simulink model "dc_motor_5hp_model2"  (R2022a)
settings: Solver=ode45  StartTime=0.0  StopTime=6  RelTol=1e-3  EnableMultiTasking=on
values from neighbouring files (symbols this model uses):
  Dm = 1e-4    (= 0.0001)    [dc_par.m]    (also in dcm_par.m = 6.04e-06)
  J = 1    [dc_par.m]    (also in dcm_par.m = 2.12e-06)
  La = 0.012    [dc_par.m]    (also in dcm_par.m = 0.12)
  Laf = 1.8    [dc_par.m]    (also in dcm_par.m = 0.0395)
  Lf = 120    [dc_par.m]
  Ra = 0.6    [dc_par.m]    (also in dcm_par.m = 7)
  Rf = 240    [dc_par.m]
  Tm = 29    [dc_par.m]    (also in dcm_par.m = 0.00353)
  Va = 240    [dc_par.m]    (also in dcm_par.m = 6)
settings Model: Creator=Jurij  LastModifiedBy=Juri
settings SolverCC: AlgebraicLoopSolver=TrustRegion
settings DataIOCC: LimitDataPoints=on  MaxDataPoints=10000  SaveFormat=Array  SignalLoggingSaveFormat=ModelDataLogs  SaveOutput=off  SaveState=on  ReturnWorkspaceOutputs=off  StateSaveName=x  TimeSaveName=t  SignalLoggingName=sigsOut
settings OptimizationCC: LifeSpan=inf
settings DebuggingCC: SaveWithParameterizedLinksMsg=none  UnderspecifiedInitializationDetection=Classic  MergeDetectMultiDrivingBlocksExec=none  SignalResolutionControl=TryResolveAllWithWarning  MultiTaskDSMMsg=warning  MultiTaskCondExecSysMsg=none  UnconnectedInputMsg=warning  UnconnectedOutputMsg=warning  UnconnectedLineMsg=warning  SFUnexpectedBacktrackingDiag=warning  SFNoUnconditionalDefaultTransitionDiag=warning  SFExecutionAtInitializationDiag=none  SFMachineParentedDataDiag=warning  ArithmeticOperatorsInVariantConditions=warning
settings HardwareCC: ProdBitPerPointer=32  ProdBitPerSizeT=32  ProdBitPerPtrDiffT=32  ProdLargestAtomicFloat=None  ProdIntDivRoundTo=Undefined  ProdEndianess=Unspecified  ProdWordSize=32  ProdHWDeviceType=32-bit Generic  TargetUnknown=on
settings ModelReferenceCC: PropagateSignalLabelsOutOfModel=off
settings SFSimCC: SimUseLocalCustomCode=off  CustomCodeUndefinedFunction=UseInterfaceOnly
settings RTWCC: RTWUseLocalCustomCode=off
settings CodeAppCC: StateflowObjectComments=on
settings GRTTargetCC: TargetLangStandard=C89/C90 (ANSI)  CombineOutputUpdateFcns=off  GRTInterface=on
settings ConfigComp: CovMetricSettings=dw  CovSaveCumulativeToWorkspaceVar=on  CovSaveSingleToWorkspaceVar=on  CovExternalEMLEnable=off

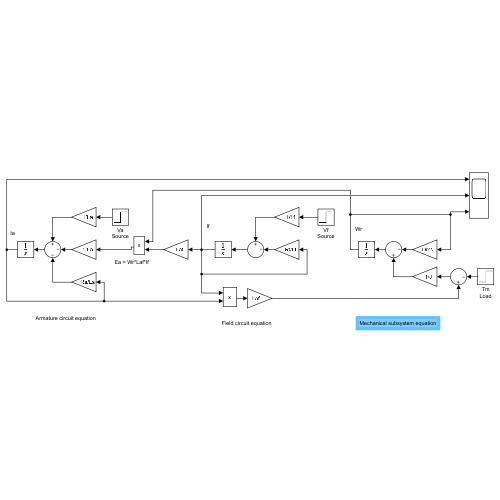
[thumbnail: Simulink's stored preview of the top-level diagram]
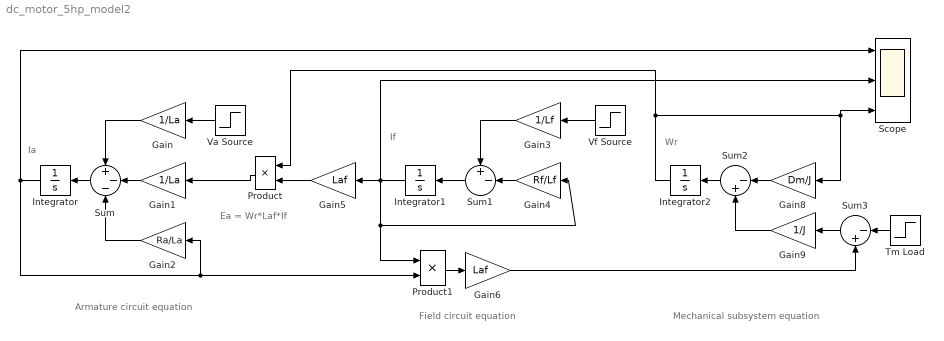
== system dc_motor_5hp_model2 ==
  note: Ia
  note: If
  note: Ea = Wr*Laf*If
  note: Wr
  note: Armature circuit equation
  note: Field circuit equation
  note: Mechanical subsystem equation
  Gain : Gain  Gain=1/La  SaturateOnIntegerOverflow=on  OutDataTypeStr=Inherit: Same as input  ParamDataTypeStr=Inherit: Same as input
  Gain1 : Gain  Gain=1/La  SaturateOnIntegerOverflow=on  OutDataTypeStr=Inherit: Same as input  ParamDataTypeStr=Inherit: Same as input
  Gain2 : Gain  Gain=Ra/La  SaturateOnIntegerOverflow=on  OutDataTypeStr=Inherit: Same as input  ParamDataTypeStr=Inherit: Same as input
  Gain3 : Gain  Gain=1/Lf  SaturateOnIntegerOverflow=on  OutDataTypeStr=Inherit: Same as input  ParamDataTypeStr=Inherit: Same as input
  Gain4 : Gain  Gain=Rf/Lf  SaturateOnIntegerOverflow=on  OutDataTypeStr=Inherit: Same as input  ParamDataTypeStr=Inherit: Same as input
  Gain5 : Gain  Gain=Laf  SaturateOnIntegerOverflow=on  OutDataTypeStr=Inherit: Same as input  ParamDataTypeStr=Inherit: Same as input
  Gain6 : Gain  Gain=Laf  SaturateOnIntegerOverflow=on  OutDataTypeStr=Inherit: Same as input  ParamDataTypeStr=Inherit: Same as input
  Gain8 : Gain  Gain=Dm/J  SaturateOnIntegerOverflow=on  OutDataTypeStr=Inherit: Same as input  ParamDataTypeStr=Inherit: Same as input
  Gain9 : Gain  Gain=1/J  SaturateOnIntegerOverflow=on  OutDataTypeStr=Inherit: Same as input  ParamDataTypeStr=Inherit: Same as input
  Integrator : Integrator
  Integrator1 : Integrator
  Integrator2 : Integrator
  Product : Product  SaturateOnIntegerOverflow=on  OutDataTypeStr=Inherit: Same as first input
  Product1 : Product  SaturateOnIntegerOverflow=on  OutDataTypeStr=Inherit: Same as first input
  Scope : Scope  NumInputPorts=3
  Sum : Sum  Inputs=+--  SaturateOnIntegerOverflow=on
  Sum1 : Sum  Inputs=+-|  SaturateOnIntegerOverflow=on
  Sum2 : Sum  Inputs=|-+  SaturateOnIntegerOverflow=on
  Sum3 : Sum  Inputs=|-+  SaturateOnIntegerOverflow=on
  Tm Load : Step  Time=4  After=Tm  SampleTime=0
  Va Source : Step  Time=2  After=Va  SampleTime=0
  Vf Source : Step  Time=0  Before=Va  After=Va  SampleTime=0
  wires:
  Gain2/1 -> Sum/3
  Gain1/1 -> Sum/2
  Gain/1 -> Sum/1
  Sum/1 -> Integrator/1
  Integrator/1 -> Gain2/1, Product1/2, Scope/1
  Va Source/1 -> Gain/1
  Gain4/1 -> Sum1/2
  Sum1/1 -> Integrator1/1
  Gain3/1 -> Sum1/1
  Vf Source/1 -> Gain3/1
  Integrator1/1 -> Gain5/1, Gain4/1, Product1/1, Scope/2
  Product/1 -> Gain1/1
  Gain5/1 -> Product/2
  Product1/1 -> Gain6/1
  Sum2/1 -> Integrator2/1
  Gain9/1 -> Sum2/2
  Gain8/1 -> Sum2/1
  Integrator2/1 -> Gain8/1, Scope/3, Product/1
  Sum3/1 -> Gain9/1
  Gain6/1 -> Sum3/2
  Tm Load/1 -> Sum3/1
